simulink model "simexample"  (R2018b)
settings: Solver=ode3  StartTime=0.0  StopTime=simTime  FixedStep=0.01  RelTol=1e-3
undefined symbols (not defined in the file): parcontroller, parmodel, reftraj
libraries: sharedtransform x2, vrlib x2, dspsigattribs x1, shared6dof x1
settings Model: Creator=duarte  LastModifiedBy=20173591
settings DataIOCC: SaveFormat=Array
settings OptimizationCC: BlockReduction=off  BooleanDataType=off  LifeSpan=inf
settings DebuggingCC: SaveWithParameterizedLinksMsg=none  SignalResolutionControl=TryResolveAllWithWarning  LibraryContextMissingDiagnostic=none  SFUnexpectedBacktrackingDiag=warning  SFNoUnconditionalDefaultTransitionDiag=warning  SFExecutionAtInitializationDiag=none
settings HardwareCC: ProdBitPerPointer=32  ProdBitPerSizeT=32  ProdBitPerPtrDiffT=32  ProdLargestAtomicFloat=None  ProdIntDivRoundTo=Undefined  ProdEndianess=Unspecified  ProdWordSize=32  ProdHWDeviceType=32-bit Generic  TargetUnknown=on
settings ModelReferenceCC: PropagateSignalLabelsOutOfModel=off
settings SFSimCC: SimUseLocalCustomCode=off
settings RTWCC: RTWUseLocalCustomCode=off
settings CodeAppCC: StateflowObjectComments=on
settings GRTTargetCC: TargetLangStandard=C89/C90 (ANSI)  GeneratePreprocessorConditionals=Disable all
settings ConfigComp: CovMetricSettings=dw  CovHtmlReporting=on  CovSaveCumulativeToWorkspaceVar=on  CovSaveSingleToWorkspaceVar=on  CovExternalEMLEnable=off  CovSFcnEnable=off

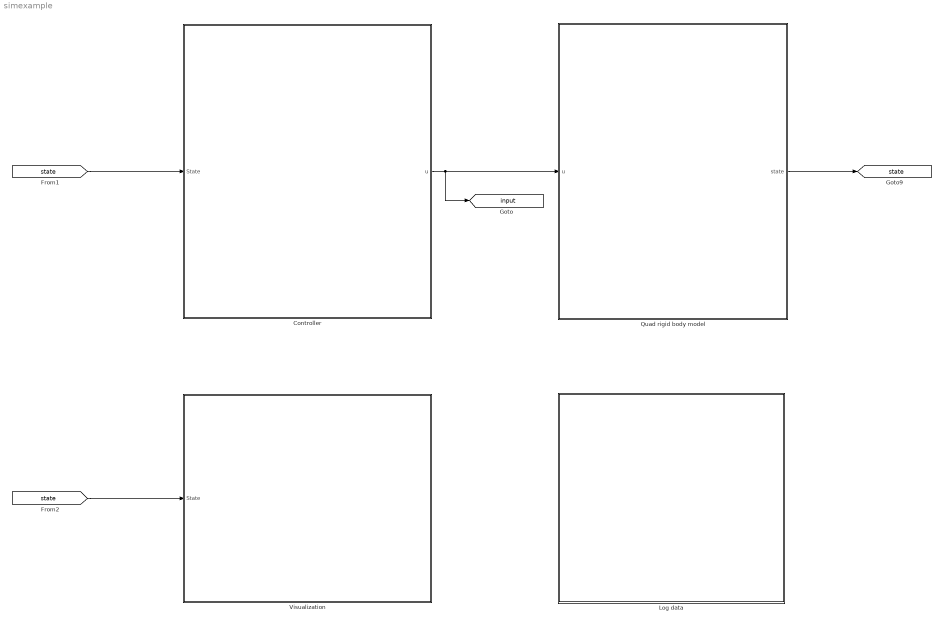
== system simexample ==
  Controller : Subsystem
  Log data : Subsystem
  Quad rigid body model : Subsystem
  Visualization : Subsystem
  tag scope: input=global, state=global
  wires:
  Quad rigid body model/1(state) -> [state]
  [state] -> Visualization/1(State)
  [state] -> Controller/1(State)
  Controller/1(u) -> [input], Quad rigid body model/1("u ")

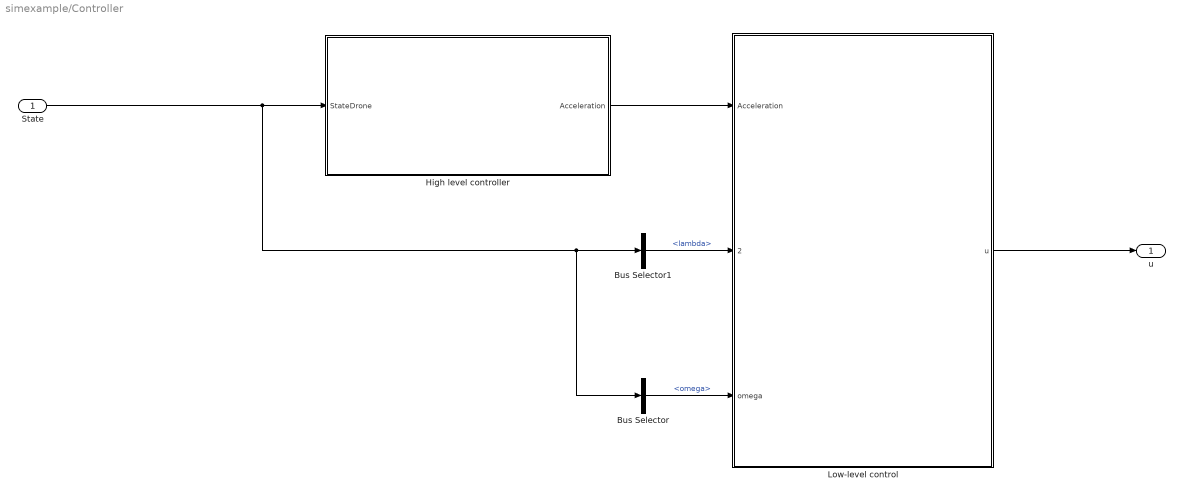
== system simexample/Controller ==
  State : Inport
  Bus Selector : BusSelector  OutputSignals=omega
  Bus Selector1 : BusSelector  OutputSignals=lambda
  High level controller : Subsystem
  Low-level control : Subsystem
  u : Outport
  wires:
  High level controller/1(Acceleration) -> Low-level control/1(Acceleration)
  Bus Selector/1 -> Low-level control/3(omega)  "<omega>"
  Bus Selector1/1 -> Low-level control/2(" ")  "<lambda>"
  State/1 -> Bus Selector/1, Bus Selector1/1, High level controller/1(StateDrone)
  Low-level control/1(u) -> u/1

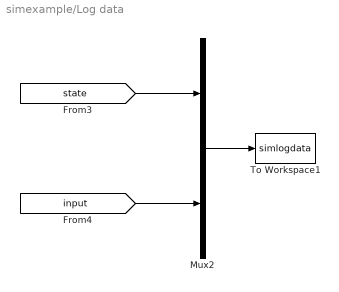
== system simexample/Log data ==
  Mux2 : Mux  Inputs=2
  To Workspace1 : ToWorkspace  VariableName=simlogdata  SaveFormat=Structure With Time  SampleTime=-1
      settings: Decimation=2
  wires:
  [input] -> Mux2/2
  Mux2/1 -> To Workspace1/1
  [state] -> Mux2/1

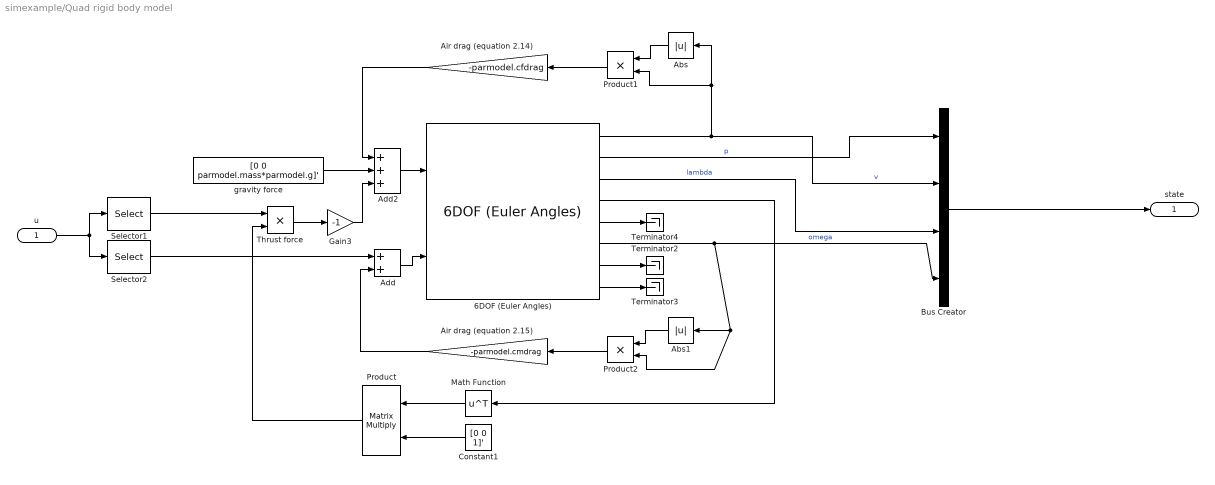
== system simexample/Quad rigid body model ==
  "u " : Inport
  6DOF (Euler Angles) : shared6dof/6DOF (Euler Angles)  units=Metric (MKS)  mtype=Fixed  rep=Euler Angles  xme_0=parmodel.pose0(1:3)  Vm_0=[0 0 0]  eul_0=[0 0 parmodel.pose0(4)]  pm_0=[0 0 0]  mass_0=parmodel.mass  mass_e=0.5  mass_f=2.0  inertia=parmodel.MomInertia  inertia_e=eye(3)  inertia_f=2*eye(3)  k_quat=1.0  vre_flag=on  abi_flag=off  aMode=aMode  xme_statename=''  Vm_statename=''  eul_statename=''  quat_statename=''  pm_statename=''  mass_statename=''
      settings: SourceProductBaseCode=AE
  Abs : Abs
  Abs1 : Abs
  Add : Sum
  Add2 : Sum  Inputs=+++
  Air drag (equation 2.14) : Gain  Gain=-parmodel.cfdrag
  Air drag (equation 2.15) : Gain  Gain=-parmodel.cmdrag
  Bus Creator : BusCreator  Inputs=4
  Constant1 : Constant  Value=[0 0 1]'
  Gain3 : Gain  Gain=-1
  Math Function : Math  Operator=transpose  SaturateOnIntegerOverflow=on
  Product : Product  Multiplication=Matrix(*)
  Product1 : Product
  Product2 : Product
  Selector1 : Selector  InputPortWidth=4  IndexOptions=Index vector (dialog)  Indices=1  OutputSizes=1
  Selector2 : Selector  InputPortWidth=4  IndexOptions=Index vector (dialog)  Indices=[2,3,4]  OutputSizes=1
  Terminator2 : Terminator
  Terminator3 : Terminator
  Terminator4 : Terminator
  Thrust force : Product
  gravity force : Constant  Value=[0 0 parmodel.mass*parmodel.g]'  VectorParams1D=off
  state : Outport
  wires:
  Constant1/1 -> Product/2
  Add2/1 -> 6DOF (Euler Angles)/1
  Math Function/1 -> Product/1
  Product/1 -> Thrust force/2
  6DOF (Euler Angles)/1 -> Product1/2, Abs/1, Bus Creator/2  "v"
  6DOF (Euler Angles)/7 -> Terminator2/1
  6DOF (Euler Angles)/8 -> Terminator3/1
  6DOF (Euler Angles)/5 -> Terminator4/1
  Thrust force/1 -> Gain3/1
  gravity force/1 -> Add2/2
  Air drag (equation 2.14)/1 -> Add2/1
  Gain3/1 -> Add2/3
  6DOF (Euler Angles)/4 -> Math Function/1
  Bus Creator/1 -> state/1
  6DOF (Euler Angles)/6 -> Bus Creator/4, Product2/2, Abs1/1  "omega"
  6DOF (Euler Angles)/3 -> Bus Creator/3  "lambda"
  6DOF (Euler Angles)/2 -> Bus Creator/1  "p"
  "u "/1 -> Selector1/1, Selector2/1
  Selector1/1 -> Thrust force/1
  Abs/1 -> Product1/1
  Product1/1 -> Air drag (equation 2.14)/1
  Product2/1 -> Air drag (equation 2.15)/1
  Abs1/1 -> Product2/1
  Air drag (equation 2.15)/1 -> Add/2
  Add/1 -> 6DOF (Euler Angles)/2
  Selector2/1 -> Add/1

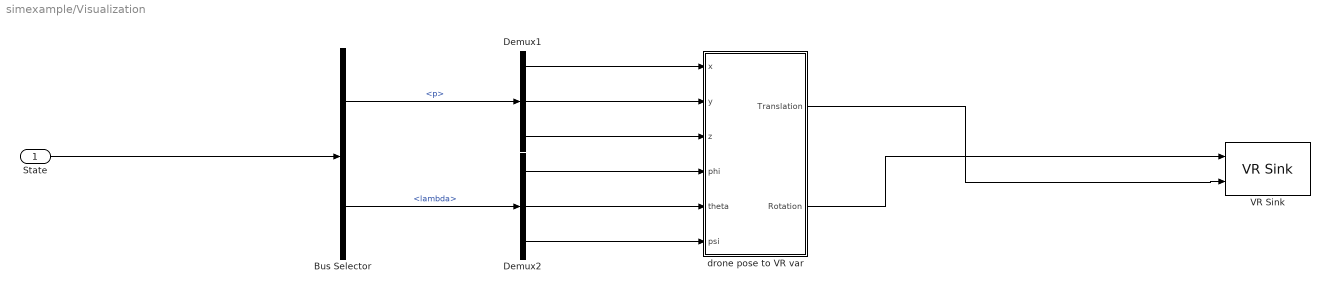
== system simexample/Visualization ==
  State : Inport
  Bus Selector : BusSelector  OutputSignals=p,lambda
  Demux1 : Demux  Outputs=3
  Demux2 : Demux  Outputs=3
  VR Sink : vrlib/VR Sink  InstantiateOnLoad=on  SampleTime=-1  ViewEnable=on  RemoteChange=off  RemoteView=off  FieldsWritten=Quad1.rotation.4.1.1.double#Quad1.translation.3.1.1.double  WorldFileName=C:\Users\20173591\OneDrive - TU Eindhoven\TU Eindhoven\Honors\Year 1\Firefly 1.0\wrl\NeutralSingleDroneLEDs.wrl  AutoView=off  VideoDimensions=[]  AllowVariableSize=off
      settings: SourceProductBaseCode=VR
  drone pose to VR var : Subsystem
  wires:
  State/1 -> Bus Selector/1
  Bus Selector/1 -> Demux1/1  "<p>"
  Bus Selector/2 -> Demux2/1  "<lambda>"
  Demux1/1 -> drone pose to VR var/1(x)
  Demux1/2 -> drone pose to VR var/2(y)
  Demux1/3 -> drone pose to VR var/3(z)
  Demux2/1 -> drone pose to VR var/4(phi)
  Demux2/2 -> drone pose to VR var/5(theta)
  Demux2/3 -> drone pose to VR var/6(psi)
  drone pose to VR var/1(Translation) -> VR Sink/2
  drone pose to VR var/2(Rotation) -> VR Sink/1

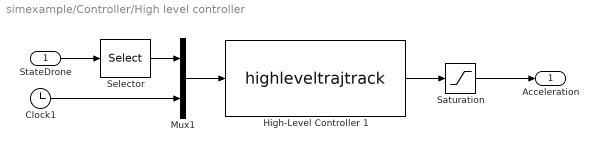
== system simexample/Controller/High level controller ==
  StateDrone : Inport
  Clock1 : Clock
  High-Level Controller 1 : S-Function  FunctionName=highleveltrajtrack  Parameters=reftraj,parcontroller  SFunctionDeploymentMode=off  EnableBusSupport=off
  Mux1 : Mux  Inputs=2
  Saturation : Saturate  UpperLimit=parcontroller.acceleration_sat  LowerLimit=-parcontroller.acceleration_sat
  Selector : Selector  InputPortWidth=12  IndexOptions=Index vector (dialog)  Indices=[1,2,3,9,4,5,6,12]  OutputSizes=1
  Acceleration : Outport
  wires:
  StateDrone/1 -> Selector/1
  Clock1/1 -> Mux1/2
  High-Level Controller 1/1 -> Saturation/1
  Saturation/1 -> Acceleration/1
  Mux1/1 -> High-Level Controller 1/1
  Selector/1 -> Mux1/1

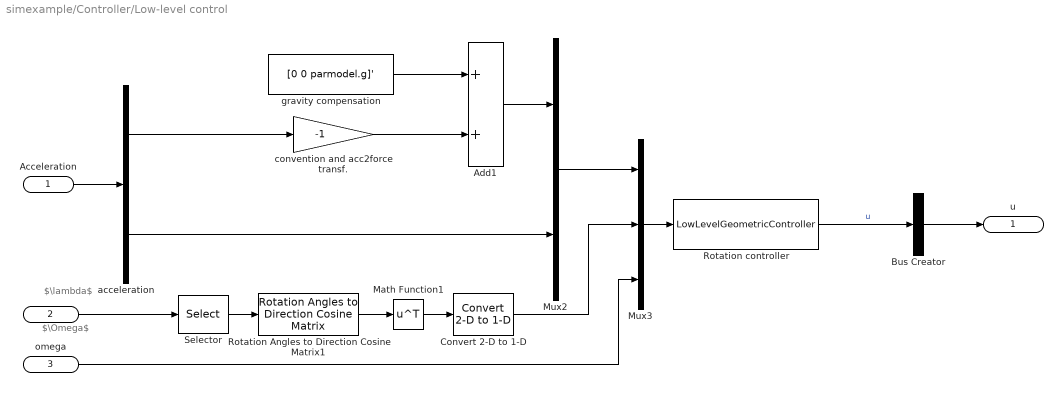
== system simexample/Controller/Low-level control ==
  note: $\Omega$
  note: $\lambda$
  Acceleration : Inport
  " " : Inport  Port=2
  omega : Inport  Port=3
  Add1 : Sum
  Bus Creator : BusCreator  Inputs=1
  Convert 2-D to 1-D : dspsigattribs/Convert 2-D to 1-D
      settings: SourceProductName=DSP System Toolbox  SourceProductBaseCode=DS
  Math Function1 : Math  Operator=transpose  SaturateOnIntegerOverflow=on
  Mux2 : Mux  Inputs=2
  Mux3 : Mux  Inputs=3
  Rotation Angles to Direction Cosine Matrix1 : sharedtransform/Rotation Angles to Direction Cosine Matrix  rotationOrder=ZYX  aMode=aMode
      settings: SourceProductBaseCode=AE
  Rotation controller : S-Function  FunctionName=LowLevelGeometricController  Parameters=parmodel, parcontroller  SFunctionDeploymentMode=off  EnableBusSupport=off
  Selector : Selector  InputPortWidth=3  IndexOptions=Index vector (dialog)  Indices=[3,2,1]  OutputSizes=1
  acceleration : Demux  Outputs=[3,1]
  convention and acc2force transf. : Gain  Gain=-1
  gravity compensation : Constant  Value=[0 0 parmodel.g]'  VectorParams1D=off
  u : Outport
  wires:
  convention and acc2force transf./1 -> Add1/2
  Add1/1 -> Mux2/1
  Mux2/1 -> Mux3/1
  gravity compensation/1 -> Add1/1
  acceleration/1 -> convention and acc2force transf./1
  Mux3/1 -> Rotation controller/1
  omega/1 -> Mux3/3
  Acceleration/1 -> acceleration/1
  acceleration/2 -> Mux2/2
  Math Function1/1 -> Convert 2-D to 1-D/1
  Convert 2-D to 1-D/1 -> Mux3/2
  Rotation Angles to Direction Cosine Matrix1/1 -> Math Function1/1
  Selector/1 -> Rotation Angles to Direction Cosine Matrix1/1
  " "/1 -> Selector/1
  Rotation controller/1 -> Bus Creator/1  "u"
  Bus Creator/1 -> u/1

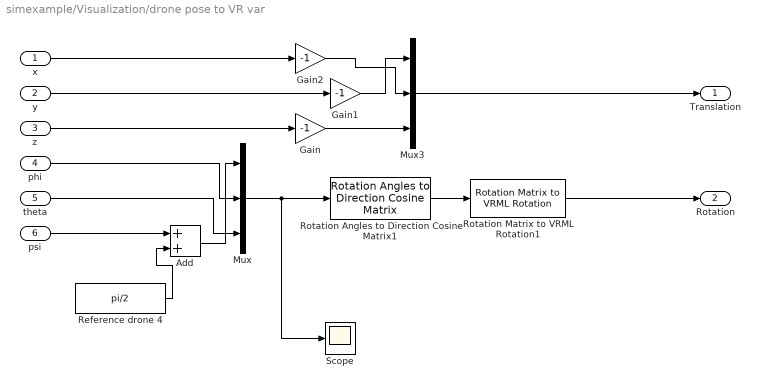
== system simexample/Visualization/drone pose to VR var ==
  x : Inport
  y : Inport  Port=2
  z : Inport  Port=3
  phi : Inport  Port=4
  theta : Inport  Port=5
  psi : Inport  Port=6
  Add : Sum
  Gain : Gain  Gain=-1
  Gain1 : Gain  Gain=-1
  Gain2 : Gain  Gain=-1
  Mux : Mux  Inputs=3
  Mux3 : Mux  Inputs=3
  Reference drone 4 : Constant  Value=pi/2
  Rotation Angles to Direction Cosine Matrix1 : sharedtransform/Rotation Angles to Direction Cosine Matrix  rotationOrder=ZYX  aMode=aMode
      settings: SourceProductBaseCode=AE
  Rotation Matrix to VRML Rotation1 : vrlib/Utilities/Rotation Matrix to VRML Rotation  maxzero=1e-12
      settings: SourceProductName=Simulink 3D Animation  SourceProductBaseCode=VR
  Scope : Scope
  Translation : Outport
  Rotation : Outport  Port=2
  wires:
  theta/1 -> Mux/3
  phi/1 -> Mux/2
  Gain/1 -> Mux3/3
  Gain1/1 -> Mux3/1
  z/1 -> Gain/1
  Gain2/1 -> Mux3/2
  x/1 -> Gain2/1
  y/1 -> Gain1/1
  Mux/1 -> Rotation Angles to Direction Cosine Matrix1/1, Scope/1
  Rotation Angles to Direction Cosine Matrix1/1 -> Rotation Matrix to VRML Rotation1/1
  psi/1 -> Add/1
  Reference drone 4/1 -> Add/2
  Add/1 -> Mux/1
  Mux3/1 -> Translation/1
  Rotation Matrix to VRML Rotation1/1 -> Rotation/1
